simulink model "sample_model"  (R2023b)
settings: Solver=VariableStepAuto  StartTime=0.0  StopTime=10.0  RelTol=1e-3
settings Model: Creator=lisjyw  LastModifiedBy=lisjyw

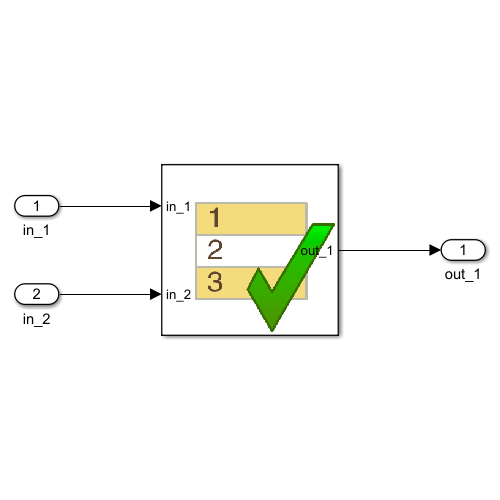
[thumbnail: Simulink's stored preview of the top-level diagram]
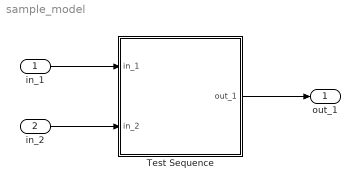
== system sample_model ==
  in_1 : Inport
  in_2 : Inport  Port=2
  Test Sequence : Test Sequence  TreatAsAtomicUnit=on
  out_1 : Outport
  wires:
  in_1/1 -> Test Sequence/1(in_1)
  in_2/1 -> Test Sequence/2(in_2)
  Test Sequence/1(out_1) -> out_1/1

== stateflow chart sample_model/Test Sequence ==
  state step_1
    out_1 = in_1 * in_2;
  (default) -> step_1
  data: in_1 input; in_2 input; out_1 output
